simulink model "VehicleDynamicsF2812Simulation"  (Simulink 6.5)
settings: Solver=FixedStepDiscrete  StartTime=0.0  StopTime=10000  RelTol=1e-3
values from neighbouring files (symbols this model uses):
  x = single(get(hObject,'Value'))    [AM.m]
undefined symbols (not defined in the file or in its folder): DiscIntNeverNeededParam
libraries: simulink x2
settings Model: Creator=Dell  LastModifiedBy=Administrator  ProdHWDeviceType=TI C2000
settings DataIOCC: SaveOutput=off  SaveTime=off
settings OptimizationCC: OptimizeModelRefInitCode=on  LifeSpan=1
settings HardwareCC: ProdBitPerChar=16  ProdBitPerInt=16  ProdIntDivRoundTo=Zero  ProdEndianess=LittleEndian  ProdWordSize=16  ProdHWDeviceType=TI C2000
settings RTWCC: SystemTargetFile=ti_c2000_ert.tlc  TemplateMakefile=ti_c2000_ert.tmf  Description=Embedded Target for TI C2000 DSP (ERT)  ProcessScript=ti_c2000_ert_make_rtw_hook
settings CodeAppCC: IgnoreCustomStorageClasses=off
settings STFCustomTargetCC: TargetFcnLib=ansi_tfl_tmw.mat  GenFloatMathFcnCalls=ANSI_C  ModelReferenceCompliant=off  CombineOutputUpdateFcns=on  ERTCustomFileBanners=on  SupportContinuousTime=off  SupportNonInlinedSFcns=off  SystemTargetFile=ti_c2000_ert.tlc
settings ERTTargetCC: TargetFcnLib=ansi_tfl_tmw.mat  GenFloatMathFcnCalls=ANSI_C  ModelReferenceCompliant=off  InlinedParameterPlacement=NonHierarchical  ERTCustomFileTemplate=example_file_process.tlc

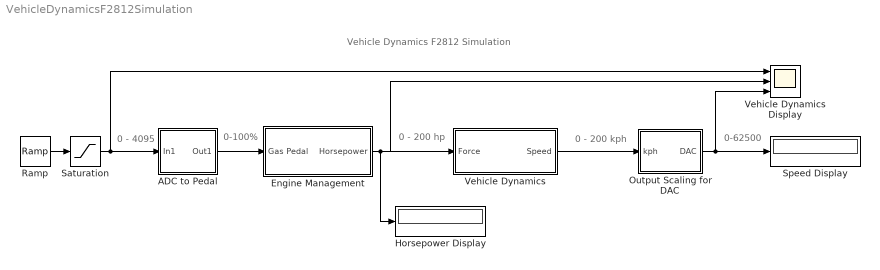
== system VehicleDynamicsF2812Simulation ==
  note: 0 - 200 kph
  note: Vehicle Dynamics F2812 Simulation
  note: 0 - 200 hp
  note: 0 - 4095
  note: 0-100%
  note: 0-62500
  ADC to Pedal : Subsystem
  Engine Management : Subsystem
  Horsepower Display : Display
  Output Scaling for DAC : Subsystem
  Ramp : simulink/Sources/Ramp  SystemSampleTime=-1  slope=0.02 * 40.95  start=0  X0=0
  Saturation : Saturate  UpperLimit=4095  LowerLimit=0
  Speed Display : Display
  "Vehicle Dynamics " : Subsystem
  Vehicle Dynamics Display : Scope  NumInputPorts=3
      settings: TimeRange=10000  YMin=0~0~0  YMax=5000~250~50000  SaveName=ScopeData2  MaxDataPoints=10000
  wires:
  "Vehicle Dynamics "/1(Speed) -> Output Scaling for DAC/1(kph)
  Engine Management/1(Horsepower) -> "Vehicle Dynamics "/1(Force), Horsepower Display/1, Vehicle Dynamics Display/2
  Saturation/1 -> ADC to Pedal/1(In1), Vehicle Dynamics Display/1
  Ramp/1 -> Saturation/1
  ADC to Pedal/1(Out1) -> Engine Management/1(Gas Pedal)
  Output Scaling for DAC/1(DAC) -> Speed Display/1, Vehicle Dynamics Display/3

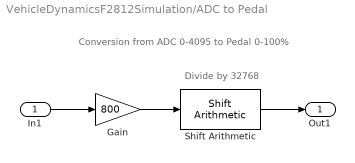
== system VehicleDynamicsF2812Simulation/ADC to Pedal ==
  note: Divide by 32768
  note: Conversion from ADC 0-4095 to Pedal 0-100%
  In1 : Inport
  Gain : Gain  Gain=800  OutDataTypeMode=Specify via dialog  OutDataType=uint(32)
  Shift Arithmetic : simulink/Logic and Bit Operations/Shift Arithmetic  SystemSampleTime=-1  nBitShiftRight=15  nBinPtShiftRight=0
  Out1 : Outport
  wires:
  In1/1 -> Gain/1
  Gain/1 -> Shift Arithmetic/1
  Shift Arithmetic/1 -> Out1/1

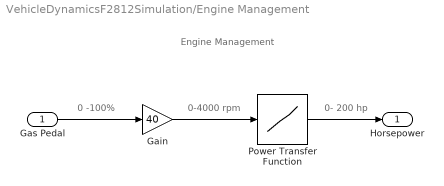
== system VehicleDynamicsF2812Simulation/Engine Management ==
  note: 0-4000 rpm
  note: 0 -100%
  note: 0- 200 hp
  note: Engine Management
  Gas Pedal : Inport
  Gain : Gain  Gain=40  ParameterDataTypeMode=Specify via dialog  ParameterDataType=uint(16)
  Power Transfer Function : Lookup  InputValues=uint16([0,500,1000,1500,2000,2500,3000,3500,4000]);  OutputValues=uint16([40,80,120,154,176,191,200,180,160]);  LookUpMeth=Interpolation-Extrapolation  OutDataTypeMode=uint16  OutDataType=sfix(16)  OutScaling=2^0  SampleTime=-1  LUTDesignTableMode=Redesign Table  LUTDesignDataSource=Block Dialog  LUTDesignFunctionName=sqrt(x)  LUTDesignUseExistingBP=on  LUTDesignRelError=0.01  LUTDesignAbsError=1e-6  SaturateOnIntegerOverflow=off  RndMeth=Floor
      settings: LockScale=off
  Horsepower : Outport
  wires:
  Gas Pedal/1 -> Gain/1
  Gain/1 -> Power Transfer Function/1
  Power Transfer Function/1 -> Horsepower/1

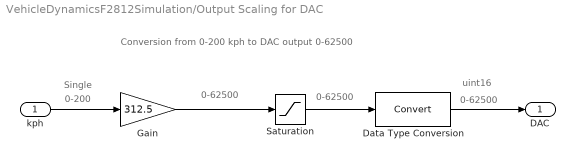
== system VehicleDynamicsF2812Simulation/Output Scaling for DAC ==
  note: 0-200
  note: 0-62500
  note: 0-62500
  note: Conversion from 0-200 kph to DAC output 0-62500
  note: Single
  note: uint16
  note: 0-62500
  kph : Inport
  Data Type Conversion : DataTypeConversion  OutDataTypeMode=uint16
  Gain : Gain  Gain=312.5
  Saturation : Saturate  UpperLimit=62500  LowerLimit=0
  DAC : Outport
  wires:
  kph/1 -> Gain/1
  Saturation/1 -> Data Type Conversion/1
  Gain/1 -> Saturation/1
  Data Type Conversion/1 -> DAC/1

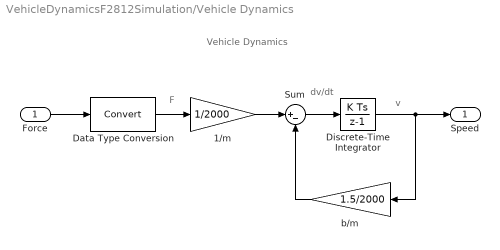
== system VehicleDynamicsF2812Simulation/Vehicle Dynamics  ==
  note: Vehicle Dynamics
  note: dv/dt
  note: v
  note: F
  Force : Inport
  1/m : Gain  Gain=1/2000
  Data Type Conversion : DataTypeConversion  OutDataTypeMode=single
  Discrete-Time Integrator : DiscreteIntegrator  ICPrevOutput=DiscIntNeverNeededParam  ICPrevScaledInput=DiscIntNeverNeededParam
  Sum : Sum  Inputs=|+-
  b/m : Gain  Orientation=left  Gain=1.5/2000
  Speed : Outport
  wires:
  Force/1 -> Data Type Conversion/1
  1/m/1 -> Sum/1
  Discrete-Time Integrator/1 -> Speed/1, b/m/1
  Sum/1 -> Discrete-Time Integrator/1
  b/m/1 -> Sum/2
  Data Type Conversion/1 -> 1/m/1
